simulink model "concatenate_test_tmp"  (Simulink 8.3)
settings: Solver=VariableStepDiscrete  StartTime=0.0  StopTime=0  MaxStep=1  RelTol=1e-3
settings Model: Creator=arnaud  LastModifiedBy=hbourbou
settings DataIOCC: SaveFormat=Structure  SignalLoggingSaveFormat=Dataset
settings DebuggingCC: UnderspecifiedInitializationDetection=Simplified  MergeDetectMultiDrivingBlocksExec=error  FrameProcessingCompatibilityMsg=error  StateNameClashWarn=none
settings GRTTargetCC: CombineOutputUpdateFcns=on  GRTInterface=off

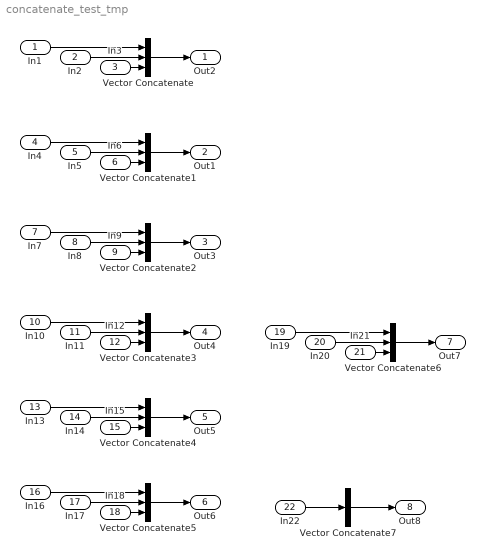
== system concatenate_test_tmp ==
  In1 : Inport
  In2 : Inport  Port=2
  In3 : Inport  Port=3
  In4 : Inport  Port=4
  In5 : Inport  Port=5  PortDimensions=5
  In6 : Inport  Port=6
  In7 : Inport  Port=7
  In8 : Inport  Port=8  PortDimensions=5
  In9 : Inport  Port=9  PortDimensions=2
  In10 : Inport  Port=10  PortDimensions=2
  In11 : Inport  Port=11  PortDimensions=5
  In12 : Inport  Port=12  PortDimensions=2
  In13 : Inport  Port=13  PortDimensions=[5 2]
  In14 : Inport  Port=14  PortDimensions=5
  In15 : Inport  Port=15  PortDimensions=5
  In16 : Inport  Port=16  PortDimensions=[5 2]
  In17 : Inport  Port=17  PortDimensions=[3 2]
  In18 : Inport  Port=18  PortDimensions=[1 2]
  In19 : Inport  Port=19  PortDimensions=2
  In20 : Inport  Port=20  PortDimensions=2
  In21 : Inport  Port=21  PortDimensions=2
  In22 : Inport  Port=22  PortDimensions=[3 2]
  Vector Concatenate : Concatenate  NumInputs=3
  Vector Concatenate1 : Concatenate  NumInputs=3
  Vector Concatenate2 : Concatenate  NumInputs=3
  Vector Concatenate3 : Concatenate  NumInputs=3  Mode=Multidimensional array
  Vector Concatenate4 : Concatenate  NumInputs=3  Mode=Multidimensional array  ConcatenateDimension=2
  Vector Concatenate5 : Concatenate  NumInputs=3  Mode=Multidimensional array
  Vector Concatenate6 : Concatenate  NumInputs=3  Mode=Multidimensional array  ConcatenateDimension=2
  Vector Concatenate7 : Concatenate  NumInputs=1  Mode=Multidimensional array  ConcatenateDimension=2
  Out2 : Outport
  Out1 : Outport  Port=2
  Out3 : Outport  Port=3
  Out4 : Outport  Port=4
  Out5 : Outport  Port=5
  Out6 : Outport  Port=6
  Out7 : Outport  Port=7
  Out8 : Outport  Port=8
  wires:
  Vector Concatenate/1 -> Out2/1
  In1/1 -> Vector Concatenate/1
  In2/1 -> Vector Concatenate/2
  In3/1 -> Vector Concatenate/3
  Vector Concatenate1/1 -> Out1/1
  In4/1 -> Vector Concatenate1/1
  In5/1 -> Vector Concatenate1/2
  In6/1 -> Vector Concatenate1/3
  Vector Concatenate2/1 -> Out3/1
  In7/1 -> Vector Concatenate2/1
  In8/1 -> Vector Concatenate2/2
  In9/1 -> Vector Concatenate2/3
  Vector Concatenate3/1 -> Out4/1
  In10/1 -> Vector Concatenate3/1
  In11/1 -> Vector Concatenate3/2
  In12/1 -> Vector Concatenate3/3
  Vector Concatenate4/1 -> Out5/1
  In13/1 -> Vector Concatenate4/1
  In14/1 -> Vector Concatenate4/2
  In15/1 -> Vector Concatenate4/3
  Vector Concatenate5/1 -> Out6/1
  In16/1 -> Vector Concatenate5/1
  In17/1 -> Vector Concatenate5/2
  In18/1 -> Vector Concatenate5/3
  Vector Concatenate6/1 -> Out7/1
  In19/1 -> Vector Concatenate6/1
  In20/1 -> Vector Concatenate6/2
  In21/1 -> Vector Concatenate6/3
  In22/1 -> Vector Concatenate7/1
  Vector Concatenate7/1 -> Out8/1
